simulink model "Stewart2"  (R2016a)
settings: Solver=FixedStepAuto  StartTime=0.0  StopTime=inf  RelTol=1e-3
libraries: arduinolib x18, neural x6
settings Model: ExtModeTrigDuration=2  Creator=costa  LastModifiedBy=costa
settings OptimizationCC: OptimizeModelRefInitCode=on  LifeSpan=1  MaxStackSize=64
settings HardwareCC: ProdBitPerInt=16  ProdBitPerPointer=16  ProdLargestAtomicFloat=None  ProdWordSize=8  ProdHWDeviceType=Atmel->AVR
settings RTWCC: SystemTargetFile=ert.tlc  HardwareBoard=Arduino Mega 2560  TemplateMakefile=ert_default_tmf  GenerateReport=on  Toolchain=Arduino AVR v1.6.1  BuildConfiguration=Faster Runs  IncludeHyperlinkInReport=on  LaunchReport=on  GenerateTraceInfo=on  GenerateTraceReport=on  GenerateTraceReportSl=on  GenerateTraceReportSf=on  GenerateTraceReportEml=on
settings CodeAppCC: ForceParamTrailComments=on  IgnoreCustomStorageClasses=off  OperatorAnnotations=on  SimulinkDataObjDesc=on  SFDataObjDesc=on  MATLABFcnDesc=on  InsertBlockDesc=on  MATLABSourceComments=on
settings ERTTargetCC: SupportContinuousTime=on  SupportVariableSizeSignals=on

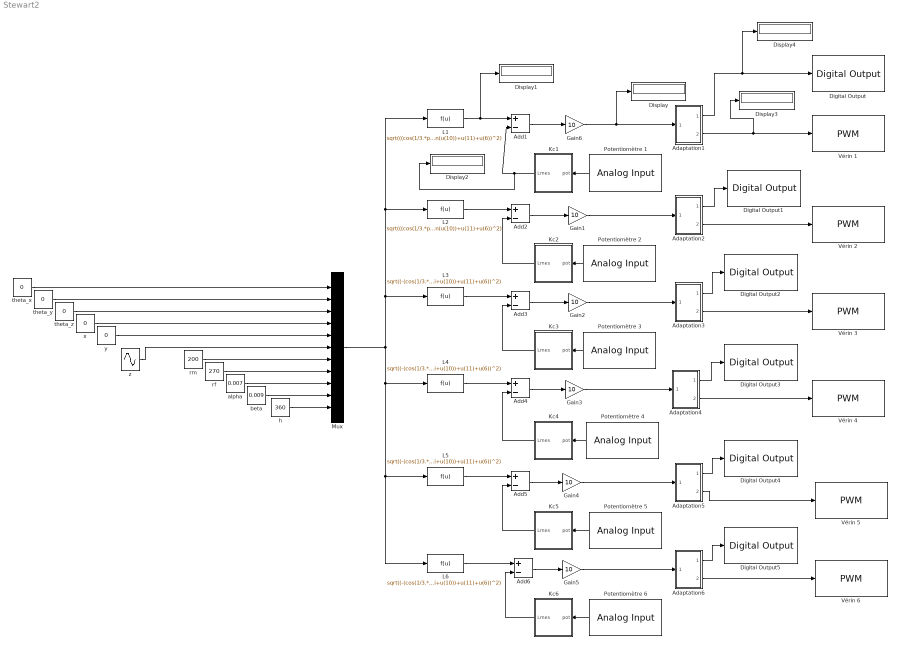
== system Stewart2 ==
  Adaptation1 : Subsystem
  Adaptation2 : Subsystem
  Adaptation3 : Subsystem
  Adaptation4 : Subsystem
  Adaptation5 : Subsystem
  Adaptation6 : Subsystem
  Add{1..6} (6 alike) : Sum  Inputs=+-
  Digital Output : arduinolib/Digital Output  pinNumber=11  blockPlatform=arduino
  Digital Output1 : arduinolib/Digital Output  pinNumber=5  blockPlatform=arduino
  Digital Output2 : arduinolib/Digital Output  pinNumber=3  blockPlatform=arduino
  Digital Output3 : arduinolib/Digital Output  pinNumber=9  blockPlatform=arduino
  Digital Output4 : arduinolib/Digital Output  pinNumber=7  blockPlatform=arduino
  Digital Output5 : arduinolib/Digital Output  pinNumber=13  blockPlatform=arduino
  Display{,1..4} (5 alike) : Display
  Gain{1..6} (6 alike) : Gain  Gain=10
  Kc1 : Subsystem
  Kc2 : Subsystem
  Kc3 : Subsystem
  Kc4 : Subsystem
  Kc5 : Subsystem
  Kc6 : Subsystem
  L1 : Fcn  Expr=sqrt(((cos(1/3.*pi+u(3))*cos(u(2))-sin(1/3.*pi+u(3))*sin(u(1))*sin(u(2)))*u(7)*cos(u(10))+sin(1/3.*pi+u(3))*cos(u(1))*u(7)*sin(u(10))-u(8)*cos(u(9))+u(4))^2+ ((sin(1/3.*pi+u(3))*cos(u(2))+cos(1/3.*pi+u(3))*sin(u(1))*sin(u(2)))*u(7)*cos(u(10))-cos(1/3.*pi+u(3))*cos(u(1))*u(7)*sin(u(10))-u(8)*sin(u(9))+u(5))^2+ (-cos(u(1))*sin(u(2))*u(7)*cos(u(10))-sin(u(1))*u(7)*sin(u(10))+u(11)+u(6))^2)
  L2 : Fcn  Expr=sqrt(((cos(1/3.*pi+u(3))*cos(u(2))-sin(1/3.*pi+u(3))*sin(u(1))*sin(u(2)))*u(7)*cos(u(10))-sin(1/3.*pi+u(3))*cos(u(1))*u(7)*sin(u(10))+u(8)*cos(1/3.*pi+u(9))+u(4))^2+ ((sin(1/3.*pi+u(3))*cos(u(2))+cos(1/3.*pi+u(3))*sin(u(1))*sin(u(2)))*u(7)*cos(u(10))+cos(1/3.*pi+u(3))*cos(u(1))*u(7)*sin(u(10))-u(8)*sin(1/3.*pi+u(9))+u(5))^2+ (-cos(u(1))*sin(u(2))*u(7)*cos(u(10))+sin(u(1))*u(7)*sin(u(10))+u(11)+u(6))^2)
  L3 : Fcn  Expr=sqrt((-(cos(1/3.*pi+u(3))*cos(u(2))-sin(1/3.*pi+u(3))*sin(u(1))*sin(u(2)))*u(7)*cos(1/3.*pi+u(10))-sin(1/3.*pi+u(3))*cos(u(1))*u(7)*sin(1/3.*pi+u(10))+u(8)*sin(1/6.*pi+u(9))+u(4))^2+(-(sin(1/3.*pi+u(3))*cos(u(2))+cos(1/3.*pi+u(3))*sin(u(1))*sin(u(2)))*u(7)*cos(1/3.*pi+u(10))+cos(1/3.*pi+u(3))*cos(u(1))*u(7)*sin(1/3.*pi+u(10))-u(8)*cos(1/6.*pi+u(9))+u(5))^2+(cos(u(1))*sin(u(2))*u(7)*cos(1/3.*pi+u(10))+sin(u(1))*u(7)*sin(1/3.*pi+u(10))+u(11)+u(6))^2)
  L4 : Fcn  Expr=sqrt((-(cos(1/3.*pi+u(3))*cos(u(2))-sin(1/3.*pi+u(3))*sin(u(1))*sin(u(2)))*u(7)*sin(1/6.*pi+u(10))-sin(1/3.*pi+u(3))*cos(u(1))*u(7)*cos(1/6.*pi+u(10))+u(8)*sin(1/6.*pi+u(9))+u(4))^2+(-(sin(1/3.*pi+u(3))*cos(u(2))+cos(1/3.*pi+u(3))*sin(u(1))*sin(u(2)))*u(7)*sin(1/6.*pi+u(10))+cos(1/3.*pi+u(3))*cos(u(1))*u(7)*cos(1/6.*pi+u(10))+u(8)*cos(1/6.*pi+u(9))+u(5))^2+(cos(u(1))*sin(u(2))*u(7)*sin(1/6.*pi+u(10))+sin(u(1))*u(7)*cos(1/6.*pi+u(10))+u(11)+u(6))^2)
  L5 : Fcn  Expr=sqrt((-(cos(1/3.*pi+u(3))*cos(u(2))-sin(1/3.*pi+u(3))*sin(u(1))*sin(u(2)))*u(7)*sin(1/6.*pi+u(10))+sin(1/3.*pi+u(3))*cos(u(1))*u(7)*cos(1/6.*pi+u(10))+u(8)*cos(1/3.*pi+u(9))+u(4))^2+(-(sin(1/3.*pi+u(3))*cos(u(2))+cos(1/3.*pi+u(3))*sin(u(1))*sin(u(2)))*u(7)*sin(1/6.*pi+u(10))-cos(1/3.*pi+u(3))*cos(u(1))*u(7)*cos(1/6.*pi+u(10))+u(8)*sin(1/3.*pi+u(9))+u(5))^2+(cos(u(1))*sin(u(2))*u(7)*sin(1/6.*pi+u(10))-sin(u(1))*u(7)*cos(1/6.*pi+u(10))+u(11)+u(6))^2)
  L6 : Fcn  Expr=sqrt((-(cos(1/3.*pi+u(3))*cos(u(2))-sin(1/3.*pi+u(3))*sin(u(1))*sin(u(2)))*u(7)*cos(1/3.*pi+u(10))+sin(1/3.*pi+u(3))*cos(u(1))*u(7)*sin(1/3.*pi+u(10))-u(8)*cos(u(9))+u(4))^2+(-(sin(1/3.*pi+u(3))*cos(u(2))+cos(1/3.*pi+u(3))*sin(u(1))*sin(u(2)))*u(7)*cos(1/3.*pi+u(10))-cos(1/3.*pi+u(3))*cos(u(1))*u(7)*sin(1/3.*pi+u(10))+u(8)*sin(u(9))+u(5))^2+(cos(u(1))*sin(u(2))*u(7)*cos(1/3.*pi+u(10))-sin(u(1))*u(7)*sin(1/3.*pi+u(10))+u(11)+u(6))^2)
  Mux : Mux  Inputs=11
  Potentiomètre 1 : arduinolib/Analog Input  pinNumber=2  sampleTime=0.001  blockPlatform=arduino
  Potentiomètre 2 : arduinolib/Analog Input  pinNumber=1  sampleTime=0.001  blockPlatform=arduino
  Potentiomètre 3 : arduinolib/Analog Input  pinNumber=0  sampleTime=0.001  blockPlatform=arduino
  Potentiomètre 4 : arduinolib/Analog Input  pinNumber=5  sampleTime=0.001  blockPlatform=arduino
  Potentiomètre 5 : arduinolib/Analog Input  pinNumber=4  sampleTime=0.001  blockPlatform=arduino
  Potentiomètre 6 : arduinolib/Analog Input  pinNumber=3  sampleTime=0.001  blockPlatform=arduino
  Vérin 1 : arduinolib/PWM  pinNumber=10  blockPlatform=arduino
  Vérin 2 : arduinolib/PWM  pinNumber=4  blockPlatform=arduino
  Vérin 3 : arduinolib/PWM  pinNumber=2  blockPlatform=arduino
  Vérin 4 : arduinolib/PWM  pinNumber=8  blockPlatform=arduino
  Vérin 5 : arduinolib/PWM  pinNumber=6  blockPlatform=arduino
  Vérin 6 : arduinolib/PWM  pinNumber=12  blockPlatform=arduino
  alpha : Constant  Value=0.007
  beta : Constant  Value=0.009
  h : Constant  Value=360
  rf : Constant  Value=270
  rm : Constant  Value=200
  theta_x : Constant  Value=0
  theta_y : Constant  Value=0
  theta_z : Constant  Value=0
  x : Constant  Value=0
  y : Constant  Value=0
  z : Sin  Amplitude=10  Frequency=3.14  SampleTime=0
  wires:
  Potentiomètre 1/1 -> Kc1/1(pot)
  h/1 -> Mux/11
  beta/1 -> Mux/10
  alpha/1 -> Mux/9
  rm/1 -> Mux/7
  rf/1 -> Mux/8
  y/1 -> Mux/5
  x/1 -> Mux/4
  theta_z/1 -> Mux/3
  theta_y/1 -> Mux/2
  theta_x/1 -> Mux/1
  L1/1 -> Display1/1, Add1/1
  Add2/1 -> Gain1/1
  Potentiomètre 2/1 -> Kc2/1(pot)
  Kc2/1(Lmes) -> Add2/2
  Add3/1 -> Gain2/1
  Potentiomètre 3/1 -> Kc3/1(pot)
  Kc3/1(Lmes) -> Add3/2
  Add4/1 -> Gain3/1
  Potentiomètre 4/1 -> Kc4/1(pot)
  Kc4/1(Lmes) -> Add4/2
  Add5/1 -> Gain4/1
  Potentiomètre 5/1 -> Kc5/1(pot)
  Kc5/1(Lmes) -> Add5/2
  Add6/1 -> Gain5/1
  Potentiomètre 6/1 -> Kc6/1(pot)
  Kc6/1(Lmes) -> Add6/2
  Mux/1 -> L3/1, L1/1, L2/1, L4/1, L5/1, L6/1
  Gain6/1 -> Display/1, Adaptation1/1(ecart)
  Adaptation1/1(sens) -> Display4/1, Digital Output/1
  Adaptation1/2(pwm) -> Display3/1, Vérin 1/1
  Adaptation2/2(pwm) -> Vérin 2/1
  Adaptation2/1(sens) -> Digital Output1/1
  Gain2/1 -> Adaptation3/1(ecart)
  Adaptation3/2(pwm) -> Vérin 3/1
  Adaptation3/1(sens) -> Digital Output2/1
  Adaptation4/2(pwm) -> Vérin 4/1
  Adaptation5/2(pwm) -> Vérin 5/1
  Adaptation5/1(sens) -> Digital Output4/1
  Adaptation4/1(sens) -> Digital Output3/1
  Adaptation6/2(pwm) -> Vérin 6/1
  Adaptation6/1(sens) -> Digital Output5/1
  Add1/1 -> Gain6/1
  Kc1/1(Lmes) -> Display2/1, Add1/2
  z/1 -> Mux/6
  L2/1 -> Add2/1
  L6/1 -> Add6/1
  L5/1 -> Add5/1
  L4/1 -> Add4/1
  L3/1 -> Add3/1
  Gain3/1 -> Adaptation4/1(ecart)
  Gain1/1 -> Adaptation2/1(ecart)
  Gain5/1 -> Adaptation6/1(ecart)
  Gain4/1 -> Adaptation5/1(ecart)

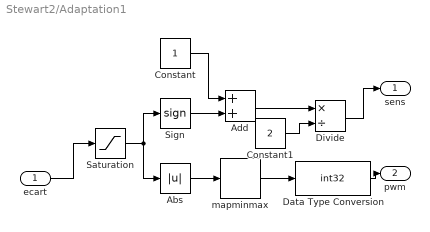
== system Stewart2/Adaptation1 ==
  ecart : Inport
  Abs : Abs
  Add : Sum
  Constant : Constant
  Constant1 : Constant  Value=2
  Data Type Conversion : DataTypeConversion  OutDataTypeStr=int32
  Divide : Product  Inputs=*/
  Saturation : Saturate  UpperLimit=200  LowerLimit=-200
  Sign : Signum
  mapminmax : neural/Processing Functions/mapminmax  xmin=0  xmax=200  ymin=0  ymax=255
  sens : Outport
  pwm : Outport  Port=2
  wires:
  ecart/1 -> Saturation/1
  Abs/1 -> mapminmax/1
  Saturation/1 -> Sign/1, Abs/1
  Sign/1 -> Add/2
  Constant/1 -> Add/1
  Add/1 -> Divide/1
  Constant1/1 -> Divide/2
  Divide/1 -> sens/1
  mapminmax/1 -> Data Type Conversion/1
  Data Type Conversion/1 -> pwm/1

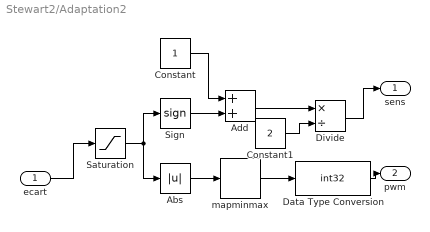
== system Stewart2/Adaptation2 ==
  ecart : Inport
  Abs : Abs
  Add : Sum
  Constant : Constant
  Constant1 : Constant  Value=2
  Data Type Conversion : DataTypeConversion  OutDataTypeStr=int32
  Divide : Product  Inputs=*/
  Saturation : Saturate  UpperLimit=200  LowerLimit=-200
  Sign : Signum
  mapminmax : neural/Processing Functions/mapminmax  xmin=0  xmax=200  ymin=0  ymax=255
  sens : Outport
  pwm : Outport  Port=2
  wires:
  ecart/1 -> Saturation/1
  Abs/1 -> mapminmax/1
  Saturation/1 -> Sign/1, Abs/1
  Sign/1 -> Add/2
  Constant/1 -> Add/1
  Add/1 -> Divide/1
  Constant1/1 -> Divide/2
  Divide/1 -> sens/1
  mapminmax/1 -> Data Type Conversion/1
  Data Type Conversion/1 -> pwm/1

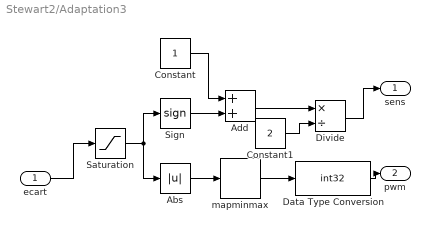
== system Stewart2/Adaptation3 ==
  ecart : Inport
  Abs : Abs
  Add : Sum
  Constant : Constant
  Constant1 : Constant  Value=2
  Data Type Conversion : DataTypeConversion  OutDataTypeStr=int32
  Divide : Product  Inputs=*/
  Saturation : Saturate  UpperLimit=200  LowerLimit=-200
  Sign : Signum
  mapminmax : neural/Processing Functions/mapminmax  xmin=0  xmax=200  ymin=0  ymax=255
  sens : Outport
  pwm : Outport  Port=2
  wires:
  ecart/1 -> Saturation/1
  Abs/1 -> mapminmax/1
  Saturation/1 -> Sign/1, Abs/1
  Sign/1 -> Add/2
  Constant/1 -> Add/1
  Add/1 -> Divide/1
  Constant1/1 -> Divide/2
  Divide/1 -> sens/1
  mapminmax/1 -> Data Type Conversion/1
  Data Type Conversion/1 -> pwm/1

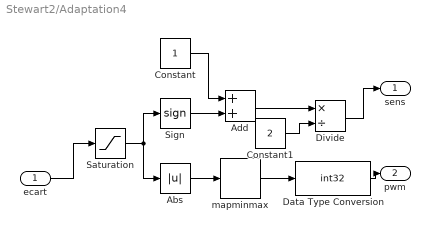
== system Stewart2/Adaptation4 ==
  ecart : Inport
  Abs : Abs
  Add : Sum
  Constant : Constant
  Constant1 : Constant  Value=2
  Data Type Conversion : DataTypeConversion  OutDataTypeStr=int32
  Divide : Product  Inputs=*/
  Saturation : Saturate  UpperLimit=200  LowerLimit=-200
  Sign : Signum
  mapminmax : neural/Processing Functions/mapminmax  xmin=0  xmax=200  ymin=0  ymax=255
  sens : Outport
  pwm : Outport  Port=2
  wires:
  ecart/1 -> Saturation/1
  Abs/1 -> mapminmax/1
  Saturation/1 -> Sign/1, Abs/1
  Sign/1 -> Add/2
  Constant/1 -> Add/1
  Add/1 -> Divide/1
  Constant1/1 -> Divide/2
  Divide/1 -> sens/1
  mapminmax/1 -> Data Type Conversion/1
  Data Type Conversion/1 -> pwm/1

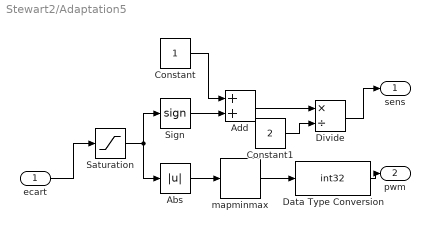
== system Stewart2/Adaptation5 ==
  ecart : Inport
  Abs : Abs
  Add : Sum
  Constant : Constant
  Constant1 : Constant  Value=2
  Data Type Conversion : DataTypeConversion  OutDataTypeStr=int32
  Divide : Product  Inputs=*/
  Saturation : Saturate  UpperLimit=200  LowerLimit=-200
  Sign : Signum
  mapminmax : neural/Processing Functions/mapminmax  xmin=0  xmax=200  ymin=0  ymax=255
  sens : Outport
  pwm : Outport  Port=2
  wires:
  ecart/1 -> Saturation/1
  Abs/1 -> mapminmax/1
  Saturation/1 -> Sign/1, Abs/1
  Sign/1 -> Add/2
  Constant/1 -> Add/1
  Add/1 -> Divide/1
  Constant1/1 -> Divide/2
  Divide/1 -> sens/1
  mapminmax/1 -> Data Type Conversion/1
  Data Type Conversion/1 -> pwm/1

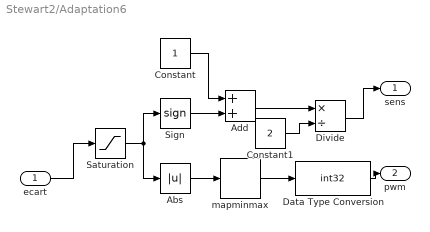
== system Stewart2/Adaptation6 ==
  ecart : Inport
  Abs : Abs
  Add : Sum
  Constant : Constant
  Constant1 : Constant  Value=2
  Data Type Conversion : DataTypeConversion  OutDataTypeStr=int32
  Divide : Product  Inputs=*/
  Saturation : Saturate  UpperLimit=200  LowerLimit=-200
  Sign : Signum
  mapminmax : neural/Processing Functions/mapminmax  xmin=0  xmax=200  ymin=0  ymax=255
  sens : Outport
  pwm : Outport  Port=2
  wires:
  ecart/1 -> Saturation/1
  Abs/1 -> mapminmax/1
  Saturation/1 -> Sign/1, Abs/1
  Sign/1 -> Add/2
  Constant/1 -> Add/1
  Add/1 -> Divide/1
  Constant1/1 -> Divide/2
  Divide/1 -> sens/1
  mapminmax/1 -> Data Type Conversion/1
  Data Type Conversion/1 -> pwm/1

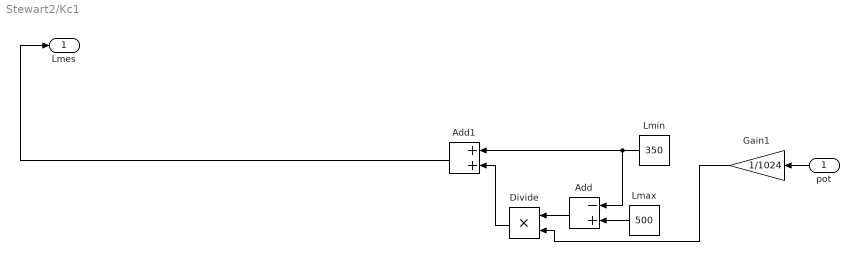
== system Stewart2/Kc1 ==
  pot : Inport
  Add : Sum  Inputs=-+
  Add1 : Sum
  Divide : Product  Inputs=**
  Gain1 : Gain  Gain=1/1024
  Lmax : Constant  Value=500
  Lmin : Constant  Value=350
  Lmes : Outport
  wires:
  Lmin/1 -> Add1/1, Add/1
  Lmax/1 -> Add/2
  Gain1/1 -> Divide/2
  Divide/1 -> Add1/2
  Add1/1 -> Lmes/1
  pot/1 -> Gain1/1
  Add/1 -> Divide/1

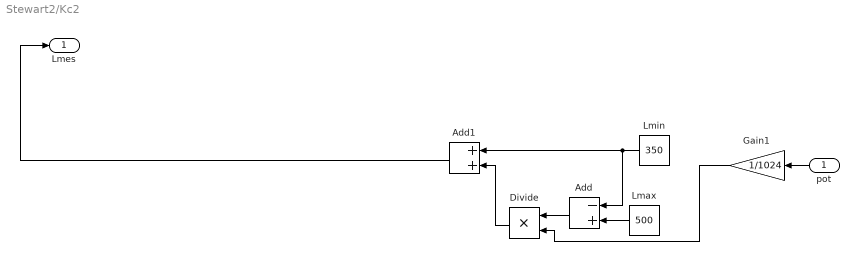
== system Stewart2/Kc2 ==
  pot : Inport
  Add : Sum  Inputs=-+
  Add1 : Sum
  Divide : Product  Inputs=**
  Gain1 : Gain  Gain=1/1024
  Lmax : Constant  Value=500
  Lmin : Constant  Value=350
  Lmes : Outport
  wires:
  Lmin/1 -> Add1/1, Add/1
  Lmax/1 -> Add/2
  Gain1/1 -> Divide/2
  Divide/1 -> Add1/2
  Add1/1 -> Lmes/1
  pot/1 -> Gain1/1
  Add/1 -> Divide/1

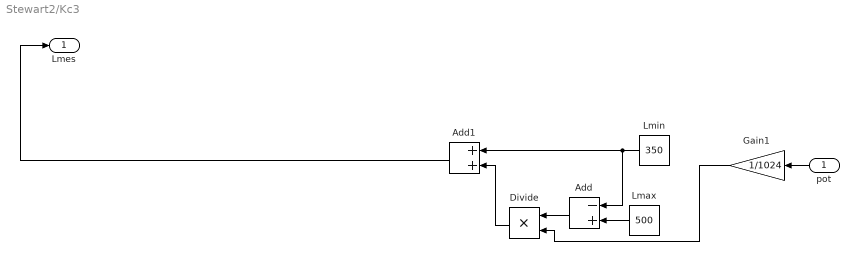
== system Stewart2/Kc3 ==
  pot : Inport
  Add : Sum  Inputs=-+
  Add1 : Sum
  Divide : Product  Inputs=**
  Gain1 : Gain  Gain=1/1024
  Lmax : Constant  Value=500
  Lmin : Constant  Value=350
  Lmes : Outport
  wires:
  Lmin/1 -> Add1/1, Add/1
  Lmax/1 -> Add/2
  Gain1/1 -> Divide/2
  Divide/1 -> Add1/2
  Add1/1 -> Lmes/1
  pot/1 -> Gain1/1
  Add/1 -> Divide/1

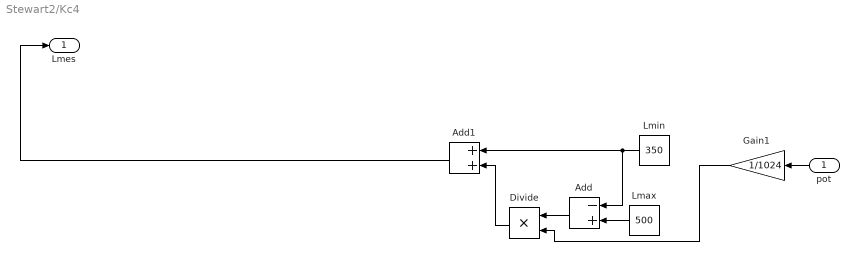
== system Stewart2/Kc4 ==
  pot : Inport
  Add : Sum  Inputs=-+
  Add1 : Sum
  Divide : Product  Inputs=**
  Gain1 : Gain  Gain=1/1024
  Lmax : Constant  Value=500
  Lmin : Constant  Value=350
  Lmes : Outport
  wires:
  Lmin/1 -> Add1/1, Add/1
  Lmax/1 -> Add/2
  Gain1/1 -> Divide/2
  Divide/1 -> Add1/2
  Add1/1 -> Lmes/1
  pot/1 -> Gain1/1
  Add/1 -> Divide/1

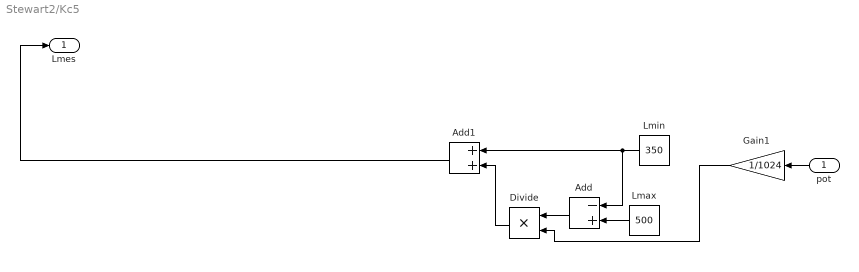
== system Stewart2/Kc5 ==
  pot : Inport
  Add : Sum  Inputs=-+
  Add1 : Sum
  Divide : Product  Inputs=**
  Gain1 : Gain  Gain=1/1024
  Lmax : Constant  Value=500
  Lmin : Constant  Value=350
  Lmes : Outport
  wires:
  Lmin/1 -> Add1/1, Add/1
  Lmax/1 -> Add/2
  Gain1/1 -> Divide/2
  Divide/1 -> Add1/2
  Add1/1 -> Lmes/1
  pot/1 -> Gain1/1
  Add/1 -> Divide/1

== system Stewart2/Kc6 ==
  pot : Inport
  Add : Sum  Inputs=-+
  Add1 : Sum
  Divide : Product  Inputs=**
  Gain1 : Gain  Gain=1/1024
  Lmax : Constant  Value=500
  Lmin : Constant  Value=350
  Lmes : Outport
  wires:
  Lmin/1 -> Add1/1, Add/1
  Lmax/1 -> Add/2
  Gain1/1 -> Divide/2
  Divide/1 -> Add1/2
  Add1/1 -> Lmes/1
  pot/1 -> Gain1/1
  Add/1 -> Divide/1
